simulink model "MON_Functional"  (R2016a)
settings: Solver=FixedStepDiscrete  StartTime=0.0  StopTime=10.0  RelTol=1e-3
undefined symbols (not defined in the file): BRAKE_PRESSURE_LO, BRAKE_PRESSURE_MAX, BRAKE_PRESSURE_MED, LO, MANUAL, MAX, MED
libraries: BSCU_lib x3, simulink x1
settings Model: Creator=jliu29  LastModifiedBy=jliu29
settings DataIOCC: LimitDataPoints=on
settings DebuggingCC: AllowSymbolicDim=off
settings ModelReferenceCC: PropagateSignalLabelsOutOfModel=off
settings RTWCC: Description=Generic Real-Time Target
settings GRTTargetCC: GeneratePreprocessorConditionals=Use local settings
settings ConfigComp: DVMode=PropertyProving  DVTestSuiteOptimization=CombinedObjectives (Nonlinear Extended)  DVAssertions=EnableAll  DVProofAssumptions=EnableAll  DVDisplayReport=off

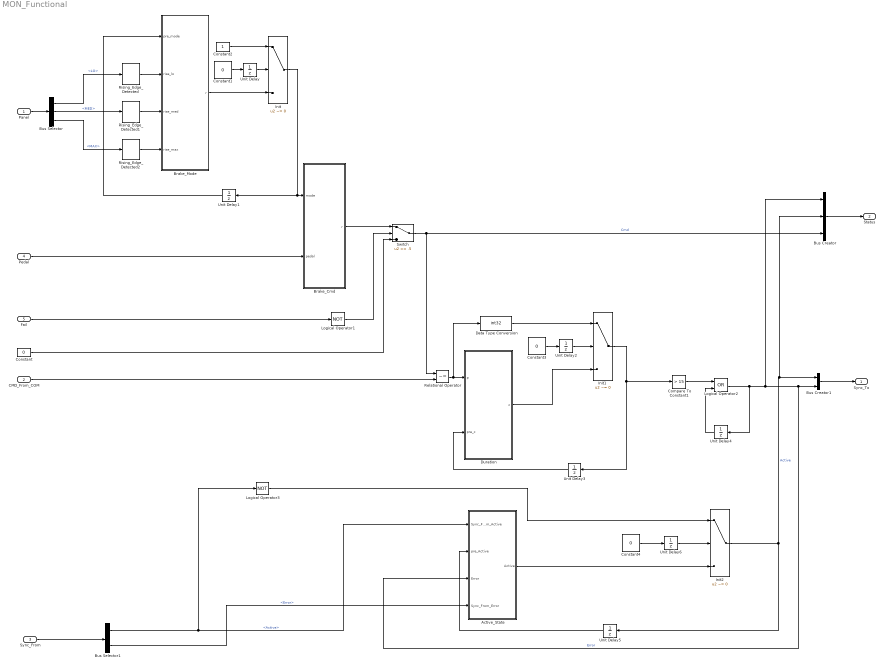
== system MON_Functional ==
  Panel : Inport  OutDataTypeStr=Bus: PanelMsgImpl
  CMD_From_COM : Inport  Port=2  OutDataTypeStr=int32
  Sync_From : Inport  Port=3  OutDataTypeStr=Bus: SyncMsgImpl
  Pedal : Inport  Port=4  OutDataTypeStr=int32
  Fail : Inport  Port=5  OutDataTypeStr=boolean
  Active_State : Stateflow chart  TreatAsAtomicUnit=on
  Brake_Cmd : Stateflow chart  TreatAsAtomicUnit=on
  Brake_Mode : Stateflow chart  TreatAsAtomicUnit=on
  Bus Creator : BusCreator  Inputs='Error','Active','Cmd'  OutDataTypeStr=Bus: ChannelStatusImpl  NonVirtualBus=on
  Bus Creator1 : BusCreator  Inputs='Active','Error'  OutDataTypeStr=Bus: SyncMsgImpl  NonVirtualBus=on
  Bus Selector : BusSelector  OutputSignals=LO,MED,MAX
  Bus Selector1 : BusSelector  OutputSignals=Active,Error
  Compare To Constant1 : simulink/Logic and Bit Operations/Compare To Constant  relop=>  const=15  OutDataTypeStr=boolean
  Constant : Constant  Value=0  OutDataTypeStr=int32
  Constant1 : Constant  DisableCoverage=on  Value=0  OutDataTypeStr=boolean
  Constant2 : Constant  OutDataTypeStr=int32
  Constant3 : Constant  DisableCoverage=on  Value=0  OutDataTypeStr=boolean
  Constant4 : Constant  DisableCoverage=on  Value=0  OutDataTypeStr=boolean
  Data Type Conversion : DataTypeConversion  OutDataTypeStr=int32
  Duration : Stateflow chart  TreatAsAtomicUnit=on
  Init : Switch  Criteria=u2 ~= 0  OutDataTypeStr=Inherit: Inherit via back propagation  ZeroCross=off  InputSameDT=on
  Init1 : Switch  Criteria=u2 ~= 0  OutDataTypeStr=Inherit: Inherit via back propagation  ZeroCross=off  InputSameDT=on
  Init2 : Switch  Criteria=u2 ~= 0  OutDataTypeStr=Inherit: Inherit via back propagation  ZeroCross=off  InputSameDT=on
  Logical Operator1 : Logic  Operator=NOT  OutDataTypeStr=boolean
  Logical Operator2 : Logic  Operator=OR  OutDataTypeStr=boolean
  Logical Operator3 : Logic  Operator=NOT  OutDataTypeStr=boolean
  Relational Operator : RelationalOperator  Operator=~=  OutDataTypeStr=boolean  ZeroCross=off  InputSameDT=on
  Rising_Edge_Detected : BSCU_lib/Rising_Edge_Detected
  Rising_Edge_Detected1 : BSCU_lib/Rising_Edge_Detected
  Rising_Edge_Detected2 : BSCU_lib/Rising_Edge_Detected
  Switch : Switch  Description=May be used within well defined functions, or functions that soley define logical expressions.  Threshold=.5  ZeroCross=off  InputSameDT=on
  Unit Delay{,1..2,6} (4 alike) : UnitDelay  InitialCondition=1  SampleTime=-1
      settings: AttributesFormatString=<Init = %<InitialCondition>>
  Unit Delay3 : UnitDelay  SampleTime=-1
      settings: AttributesFormatString=<Init = %<InitialCondition>>
  Unit Delay4 : UnitDelay  SampleTime=-1
      settings: AttributesFormatString=<Init = %<InitialCondition>>
  Unit Delay5 : UnitDelay  SampleTime=-1
      settings: AttributesFormatString=<Init = %<InitialCondition>>
  Sync_To : Outport  OutDataTypeStr=Bus: SyncMsgImpl
  Status : Outport  Port=2  OutDataTypeStr=Bus: ChannelStatusImpl
  wires:
  Brake_Mode/1(r) -> Init/3
  Init/1 -> Unit Delay1/1, Brake_Cmd/1(mode)
  Panel/1 -> Bus Selector/1
  Bus Selector/1 -> Rising_Edge_Detected/1  "<LO>"
  Bus Selector/2 -> Rising_Edge_Detected1/1  "<MED>"
  Bus Selector/3 -> Rising_Edge_Detected2/1  "<MAX>"
  Rising_Edge_Detected/1 -> Brake_Mode/2(rise_lo)
  Rising_Edge_Detected1/1 -> Brake_Mode/3(rise_med)
  Rising_Edge_Detected2/1 -> Brake_Mode/4(rise_max)
  Pedal/1 -> Brake_Cmd/2(pedal)
  Bus Creator/1 -> Status/1
  Fail/1 -> Logical Operator1/1
  Brake_Cmd/1(r) -> Switch/1
  Logical Operator1/1 -> Switch/2
  Switch/1 -> Bus Creator/3, Relational Operator/1  "Cmd"
  Constant/1 -> Switch/3
  CMD_From_COM/1 -> Relational Operator/2
  Relational Operator/1 -> Data Type Conversion/1, Duration/1(p)
  Logical Operator2/1 -> Unit Delay4/1, Bus Creator/1, Active_State/3(Error), Bus Creator1/2  "Error"
  Compare To Constant1/1 -> Logical Operator2/1
  Bus Creator1/1 -> Sync_To/1
  Sync_From/1 -> Bus Selector1/1
  Bus Selector1/1 -> Logical Operator3/1, Active_State/1(Sync_From_Active)  "<Active>"
  Bus Selector1/2 -> Active_State/4(Sync_From_Error)  "<Error>"
  Unit Delay/1 -> Init/2
  Constant1/1 -> Unit Delay/1
  Constant2/1 -> Init/1
  Duration/1(c) -> Init1/3
  Unit Delay2/1 -> Init1/2
  Constant3/1 -> Unit Delay2/1
  Data Type Conversion/1 -> Init1/1
  Init1/1 -> Compare To Constant1/1, Unit Delay3/1
  Active_State/1(Active) -> Init2/3
  Constant4/1 -> Unit Delay6/1
  Logical Operator3/1 -> Init2/1
  Init2/1 -> Unit Delay5/1, Bus Creator/2, Bus Creator1/1  "Active"
  Unit Delay1/1 -> Brake_Mode/1(pre_mode)
  Unit Delay3/1 -> Duration/2(pre_c)
  Unit Delay4/1 -> Logical Operator2/2
  Unit Delay5/1 -> Active_State/2(pre_Active)
  Unit Delay6/1 -> Init2/2

== stateflow chart MON_Functional/Brake_Cmd ==
  (default) -> (junction 4789)
  (junction 4789) -> (junction 4790) [order 1] : [mode == LO]
  (junction 4789) -> (junction 4791) [order 2]
  (junction 4790) -> (junction 4798) : {
      | r = BRAKE_PRESSURE_LO;
      | }
  (junction 4791) -> (junction 4792) [order 1] : [mode == MED ]
  (junction 4791) -> (junction 4793) [order 2]
  (junction 4792) -> (junction 4797) : {
      | r = BRAKE_PRESSURE_MED;
      | }
  (junction 4793) -> (junction 4794) [order 1] : [mode == MAX]
  (junction 4793) -> (junction 4800) [order 2]
  (junction 4794) -> (junction 4796) : {
      | r = BRAKE_PRESSURE_MAX;
      | }
  (junction 4800) -> (junction 4795) : {
      | r = pedal;
      | }
  (junction 4796) -> (junction 4795)
  (junction 4797) -> (junction 4796)
  (junction 4798) -> (junction 4797)
  (junction 4795) -> (junction 4799)
  data: mode input int32; pedal input int32; r output int32; MANUAL parameter =1; LO parameter =2; MED parameter =3; MAX parameter =4; BRAKE_PRESSURE_LO parameter; BRAKE_PRESSURE_MAX parameter; BRAKE_PRESSURE_MED parameter

== stateflow chart MON_Functional/Brake_Mode ==
  (default) -> (junction 4789)
  (junction 4789) -> (junction 4790) [order 1] : [  ((pre_mode == LO) && rise_lo) || ...
      |    ((pre_mode == MED) && rise_med) || ...
      |    ((pre_mode == MAX) && rise_max)
      | ]
  (junction 4789) -> (junction 4791) [order 2]
  (junction 4790) -> (junction 4798) : {
      | r = MANUAL;
      | }
  (junction 4791) -> (junction 4792) [order 1] : [  (pre_mode != LO) && rise_lo ]
  (junction 4791) -> (junction 4793) [order 2]
  (junction 4792) -> (junction 4797) : {
      | r = LO;
      | }
  (junction 4793) -> (junction 4794) [order 1] : [ (pre_mode != MED) && rise_med ]
  (junction 4793) -> (junction 4800) [order 2]
  (junction 4794) -> (junction 4796) : {
      | r = MED;
      | }
  (junction 4800) -> (junction 4808) [order 1] : [ (pre_mode != MAX) && rise_max ]
  (junction 4800) -> (junction 4795) [order 2] : {
      | r = pre_mode;
      | }
  (junction 4808) -> (junction 4810) : {
      | r = MAX;
      | }
  (junction 4810) -> (junction 4795)
  (junction 4796) -> (junction 4810)
  (junction 4797) -> (junction 4796)
  (junction 4798) -> (junction 4797)
  (junction 4795) -> (junction 4799)
  data: pre_mode input int32; rise_lo input boolean; rise_med input boolean; rise_max input boolean; r output int32; MANUAL parameter =1; LO parameter =2; MED parameter =3; MAX parameter =4

== stateflow chart MON_Functional/Duration ==
  (default) -> (junction 4827)
  (junction 4827) -> (junction 4828) [order 1] : [p]
  (junction 4827) -> (junction 4829) [order 2] : {c = 0;}
  (junction 4828) -> (junction 4830) : {c = pre_c+1;}
  (junction 4830) -> (junction 4829)
  (junction 4829) -> (junction 4831)
  data: p input boolean; c output int32; pre_c input int32

== stateflow chart MON_Functional/Active_State ==
  (default) -> (junction 4848)
  (junction 4848) -> (junction 4849) [order 1] : [Error]
  (junction 4848) -> (junction 4850) [order 2]
  (junction 4849) -> (junction 4857) : {Active = false;}
  (junction 4850) -> (junction 4851) [order 1] : [pre_Active && Sync_From_Active && (! Sync_From_Error) && (! Primary_Side) ]
  (junction 4850) -> (junction 4852) [order 2]
  (junction 4851) -> (junction 4856) : {Active = false;}
  (junction 4852) -> (junction 4853) [order 1] : [(!pre_Active) && ( (!Sync_From_Active) || Sync_From_Error)]
  (junction 4852) -> (junction 4854) [order 2] : {Active = pre_Active;}
  (junction 4853) -> (junction 4855) : {Active = true;}
  (junction 4855) -> (junction 4854)
  (junction 4856) -> (junction 4855)
  (junction 4857) -> (junction 4856)
  (junction 4854) -> (junction 4858)
  data: Sync_From_Active input boolean; Active output boolean; pre_Active input boolean; Error input boolean; Sync_From_Error input boolean; Primary_Side parameter
